simulink model "Degradation_Trial_1"  (R2022a)
settings: Solver=VariableStepAuto  StartTime=0.0  StopTime=500  RelTol=1e-3
libraries: nesl_utility x24, fl_lib x8
settings Model: Creator=YASH PATHAK  LastModifiedBy=YASH PATHAK

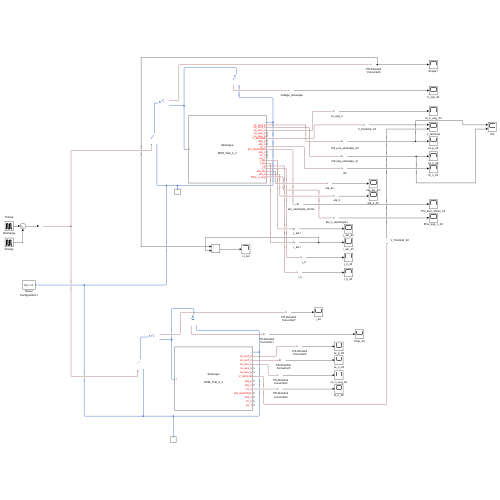
[thumbnail: Simulink's stored preview of the top-level diagram]
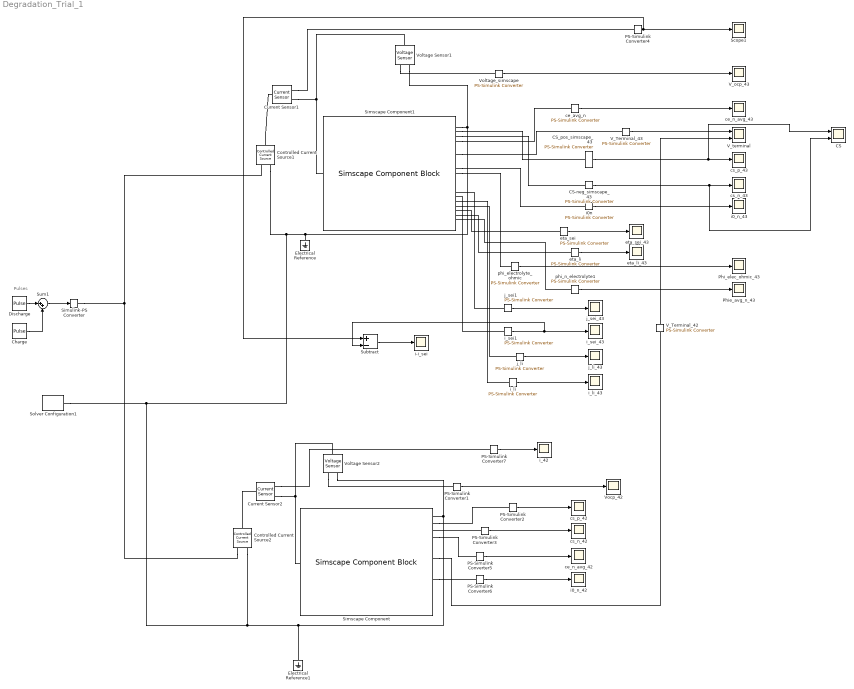
== system Degradation_Trial_1 ==
  note: Pulses
  CS : Scope  NumInputPorts=2
  CS-neg_simscape_43 : nesl_utility/PS-Simulink Converter  PhysicalDomain=network_engine_domain  SubClassName=ps_output  LeftPortType=input  RightPortType=output  PseudoPeriodic=off  Frequencies=[]  VectorFormat=inherit  Unit=inherit  AffineConversion=off
      settings: SourceProductBaseCode=SS,PW,VE
  CS_pos_simscape_43 : nesl_utility/PS-Simulink Converter  PhysicalDomain=network_engine_domain  SubClassName=ps_output  LeftPortType=input  RightPortType=output  PseudoPeriodic=off  Frequencies=[]  VectorFormat=inherit  Unit=inherit  AffineConversion=off
      settings: SourceProductBaseCode=SS,PW,VE
  Charge : DiscretePulseGenerator  PulseType=Time based  Amplitude=-25  Period=100  PulseWidth=25  PhaseDelay=75
  Controlled Current Source1 : fl_lib/Electrical/Electrical Sources/Controlled Current Source
      settings: SourceProductBaseCode=PW,SS,VE
  Controlled Current Source2 : fl_lib/Electrical/Electrical Sources/Controlled Current Source
      settings: SourceProductBaseCode=PW,SS,VE
  Current Sensor1 : fl_lib/Electrical/Electrical Sensors/Current Sensor
      settings: SourceProductBaseCode=PW,SS,VE
  Current Sensor2 : fl_lib/Electrical/Electrical Sensors/Current Sensor
      settings: SourceProductBaseCode=PW,SS,VE
  Discharge : DiscretePulseGenerator  PulseType=Time based  Amplitude=5  Period=100  PulseWidth=25  PhaseDelay=25
  Electrical Reference : fl_lib/Electrical/Electrical Elements/Electrical Reference
      settings: SourceProductBaseCode=PW,SS,VE
  Electrical Reference1 : fl_lib/Electrical/Electrical Elements/Electrical Reference
      settings: SourceProductBaseCode=PW,SS,VE
  PS-Simulink Converter{1..7} (7 alike) : nesl_utility/PS-Simulink Converter  PhysicalDomain=network_engine_domain  SubClassName=ps_output  LeftPortType=input  RightPortType=output  PseudoPeriodic=off  Frequencies=[]  VectorFormat=inherit  Unit=inherit  AffineConversion=off
      settings: SourceProductBaseCode=SS,PW,VE
  Phi_elec_ohmic_43 : Scope
  Phie_avg_n_43 : Scope
  Scope1 : Scope
  Simscape Component : SimscapeComponentBlock  SourceFile=SPM_Trial_4_2  ComponentPath=SPM_Trial_4_2  ComponentVariants="[\"SPM_Trial_4_2\"]"  ComponentVariantNames="[\"SPM_Trial_4_2\"]"  ClassName=SPM_Trial_4_2  SchemaVersion=1  nr=50  nn=50  ns=25  np=50  Rp=3.5e-06 m  Rn=2.5e-06 m  Ds_p=8e-15 m^2/s  Ds_n=5e-15 m^2/s  D_e=5.35e-10 m^2/s  D_e1=5.35e-10  SOC_0=0.1  brugg=1.5  t_plus=0.38  tf=0.62  ce_init=1000 mol/m^3  ce_init_unitless=1000  kappa=1.3 S/m  k0_n=1.061e-6 / 96485  k0_p=4.824e-6 / 96485  kt_n=1 * 0.0250 V*m^2/A  kt_p=0 * 300e-4 V*m^2/A  x100_percent_n=0.8292  x0_percent_n=3.5506e-04  y0_percent_p=0.8941  y100_percent_p=0.0335  del_p=6.7e-05 m  del_n=6.2e-05 m  del_s=1.2e-05 m  del_p1=6.7e-05  del_n1=6.2e-05  del_s1=1.2e-05  cs_max_p=35380 mol/m^3  cs_max_p_unitless=35380  cs_max_n=28746 mol/m^3  cs_max_n_unitless=28746  epsilon_e_p=0.3  epsilon_e_n=0.3  epsilon_e_s=0.4  Active_Area=0.205 m^2  Faradays=96485 C/mol  T=273.15 + 25  R=8.3145  Cap_n=6.0272 C  Cap_p=5.8050 C  i_specify=off  i_priority=None  i=0 A  i_nominal_specify=off  i_nominal_unit=A  i_nominal_value=1  v_specify=off  v_priority=None  v=0 V  v_nominal_specify=off  v_nominal_unit=V  v_nominal_value=1  UP_specify=off  UP_priority=None  UP=0  UP_nominal_specify=off  UP_nominal_unit=1  UP_nominal_value=1  UN_specify=off  UN_priority=None  UN=0  UN_nominal_specify=off  UN_nominal_unit=1  UN_nominal_value=1  V_ocp_specify=off  V_ocp_priority=None  V_ocp=0  V_ocp_nominal_specify=off  V_ocp_nominal_unit=1  V_ocp_nominal_value=1  j_n_specify=off  j_n_priority=None  j_n=0  j_n_nominal_specify=off  j_n_nominal_unit=1  j_n_nominal_value=1  j_p_specify=off  j_p_priority=None  j_p=0  j_p_nominal_specify=off  j_p_nominal_unit=1  j_p_nominal_value=1  i0_p_specify=off  i0_p_priority=None  i0_p=0  i0_p_nominal_specify=off  i0_p_nominal_unit=1  i0_p_nominal_value=1  Vr_p_specify=off  Vr_p_priority=None  Vr_p=0  Vr_p_nominal_specify=off  Vr_p_nominal_unit=1  Vr_p_nominal_value=1  x_specify=off  x_priority=None  x=0  x_nominal_specify=off  x_nominal_unit=1  x_nominal_value=1  y_specify=off  y_priority=None  y=0  y_nominal_specify=off  y_nominal_unit=1  y_nominal_value=1
      settings: CopyFcn=simscape.engine.sli.internal.componentblockcallback(gcbh,'COPY')  PreCopyFcn=simscape.engine.sli.internal.componentblockcallback(gcbh,'PRECOPY')  PreDeleteFcn=simscape.engine.sli.internal.componentblockcallback(gcbh,'PREDELETE')  InternalSimscapePortConfiguration="{\"Bottom\":[],\"Left\":[{\"id\":\"p\",\"label\":\"+\",\"type\":\"foundation.electrical.electrical\"}],\"Right\":[{\"id\":\"n\",\"label\":\"-\",\"type\":\"foundation.electrical.electrical\"},{\"id\":\"cs_surf_p\",\"label\":\"cs_surf_p\",\"type\":\"output\"},{\"id\":\"cs_surf_n\",\"label\":\"cs_surf_n\",\"type\":\"output\"},{\"id\":\"ce_ave_n\",\"label\":\"ce_ave_n\",\"type\":\"output\"},{\"id\":\"ce_ave_s\",\"label\":\"ce_ave_s\",\"type\":\"output\"},{\"id\":\"ce_ave_p\",\"label\":\"ce_ave_p\",\"type\":\"output\"},{\"id\":\"V_terminal\",\"label\":\"V_terminal\",\"type\":\"output\"},{\"id\":\"eta_p\",\"label\":\"eta_p\",\"type\":\"output\"},{\"id\":\"eta_n\",\"label\":\"eta_n\",\"type\":\"output\"},{\"id\":\"i0_n\",\"label\":\"i0_n\",\"type\":\"output\"},{\"id\":\"phi_electrolyte\",\"label\":\"phi_electrolyte\",\"type\":\"output\"},{\"id\":\"eta_c\",\"label\":\"eta_c\",\"type\":\"output\"},{\"id\":\"Vr_n\",\"label\":\"Vr_n\",\"type\":\"output\"},{\"id\":\"ce_1\",\"label\":\"ce_1\",\"type\":\"output\"}],\"Top\":[]}"
      mask Type: Two-port electrical component
  Simscape Component1 : SimscapeComponentBlock  SourceFile=SPM_Trial_4_3  ComponentPath=SPM_Trial_4_3  ComponentVariants="[\"SPM_Trial_4_3\"]"  ComponentVariantNames="[\"SPM_Trial_4_3\"]"  ClassName=SPM_Trial_4_3  SchemaVersion=1  nr=50  nn=50  ns=25  np=50  Rp=3.5e-06 m  Rn=2.5e-06 m  Ds_p=8e-15 m^2/s  Ds_n=5e-15 m^2/s  del_p=6.7e-05 m  del_n=6.2e-05 m  del_s=1.2e-05 m  del_p1=6.7e-05  del_n1=6.2e-05  del_s1=1.2e-05  cs_max_p=35380 mol/m^3  cs_max_p_unitless=35380  cs_max_n=28746 mol/m^3  cs_max_n_unitless=28746  epsilon_e_p=0.3  epsilon_e_n=0.3  epsilon_e_s=0.4  D_e=5.35e-10 m^2/s  D_e1=5.35e-10  brugg=1.5  t_plus=0.38  ce_init=1000 mol/m^3  ce_init_unitless=1000  kappa=1.3 S/m  k0_n=1.061e-6 / 96485  k0_p=4.824e-6 / 96485  kt_n=1 * 0.0250 V*m^2/A  kt_p=0 * 300e-4 V*m^2/A  x100_percent_n=0.8292  x0_percent_n=3.5506e-04  y0_percent_p=0.8941  y100_percent_p=0.0335  Faradays=96485 C/mol  T=273.15 + 25  R=8.3145  Cap_n=6.0272 C  Cap_p=5.8050 C  Active_Area=0.205 m^2  SOC_0=0.1  U_sei=0 V  i0pl=0.001 A/m^2  del_sei_init=5e-9 m  D_ec=2e-18 m^2/s  c_ec0=4541 mol/m^3  M_sei=0.162 kg/mol  rho_sei=1690 kg/m^3  k0_sei=1e-12 m/s  k_sei=5e-6 S/m  M_li=6.94e-3 kg/mol  rho_li=534 kg/m^3  i_specify=off  i_priority=None  i=0 A  i_nominal_specify=off  i_nominal_unit=A  i_nominal_value=1  v_specify=off  v_priority=None  v=0 V  v_nominal_specify=off  v_nominal_unit=V  v_nominal_value=1  UP_specify=off  UP_priority=None  UP=0  UP_nominal_specify=off  UP_nominal_unit=1  UP_nominal_value=1  UN_specify=off  UN_priority=None  UN=0  UN_nominal_specify=off  UN_nominal_unit=1  UN_nominal_value=1  V_ocp_specify=off  V_ocp_priority=None  V_ocp=0  V_ocp_nominal_specify=off  V_ocp_nominal_unit=1  V_ocp_nominal_value=1  Vr_p_specify=off  Vr_p_priority=None  Vr_p=0  Vr_p_nominal_specify=off  Vr_p_nominal_unit=1  Vr_p_nominal_value=1  j_n_specify=off  j_n_priority=None  j_n=0  j_n_nominal_specify=off  j_n_nominal_unit=1  j_n_nominal_value=1  j_p_specify=off  j_p_priority=None  j_p=0  j_p_nominal_specify=off  j_p_nominal_unit=1  j_p_nominal_value=1  i0_p_specify=off  i0_p_priority=None  i0_p=0  i0_p_nominal_specify=off  i0_p_nominal_unit=1  i0_p_nominal_value=1  x_specify=off  x_priority=None  x=0  x_nominal_specify=off  x_nominal_unit=1  x_nominal_value=1  y_specify=off  y_priority=None  y=0  y_nominal_specify=off  y_nominal_unit=1  y_nominal_value=1  Li_loss_specify=off  Li_loss_priority=None  Li_loss=0 mol  Li_loss_nominal_specify=off  Li_loss_nominal_unit=mol  Li_loss_nominal_value=1  Li_plated_specify=off  Li_plated_priority=None  Li_plated=0 mol  Li_plated_nominal_specify=off  Li_plated_nominal_unit=mol  Li_plated_nominal_value=1  Q_loss_specify=off  Q_loss_priority=None  Q_loss=0 A*hr  Q_loss_nominal_specify=off  Q_loss_nominal_unit=A*hr  Q_loss_nominal_value=1  soc_loss_specify=off  soc_loss_priority=None  soc_loss=0  soc_loss_nominal_specify=off  soc_loss_nominal_unit=1  soc_loss_nominal_value=1
      settings: CopyFcn=simscape.engine.sli.internal.componentblockcallback(gcbh,'COPY')  PreCopyFcn=simscape.engine.sli.internal.componentblockcallback(gcbh,'PRECOPY')  PreDeleteFcn=simscape.engine.sli.internal.componentblockcallback(gcbh,'PREDELETE')  InternalSimscapePortConfiguration="{\"Bottom\":[],\"Left\":[{\"id\":\"p\",\"label\":\"+\",\"type\":\"foundation.electrical.electrical\"}],\"Right\":[{\"id\":\"n\",\"label\":\"-\",\"type\":\"foundation.electrical.electrical\"},{\"id\":\"cs_surf_p\",\"label\":\"cs_surf_p\",\"type\":\"output\"},{\"id\":\"cs_surf_n\",\"label\":\"cs_surf_n\",\"type\":\"output\"},{\"id\":\"ce_ave_n\",\"label\":\"ce_ave_n\",\"type\":\"output\"},{\"id\":\"ce_ave_s\",\"label\":\"ce_ave_s\",\"type\":\"output\"},{\"id\":\"ce_ave_p\",\"label\":\"ce_ave_p\",\"type\":\"output\"},{\"id\":\"V_terminal\",\"label\":\"V_terminal\",\"type\":\"output\"},{\"id\":\"eta_p\",\"label\":\"eta_p\",\"type\":\"output\"},{\"id\":\"eta_n\",\"label\":\"eta_n\",\"type\":\"output\"},{\"id\":\"i0_n\",\"label\":\"i0_n\",\"type\":\"output\"},{\"id\":\"phi_electrolyte\",\"label\":\"phi_electrolyte\",\"type\":\"output\"},{\"id\":\"eta_c\",\"label\":\"eta_c\",\"type\":\"output\"},{\"id\":\"Vr_n\",\"label\":\"Vr_n\",\"type\":\"output\"},{\"id\":\"ce_1\",\"label\":\"ce_1\",\"type\":\"output\"},{\"id\":\"j_sei\",\"label\":\"j_sei\",\"type\":\"output\"},{\"id\":\"i_sei\",\"label\":\"i_sei\",\"type\":\"output\"},{\"id\":\"i_li\",\"label\":\"i_li\",\"type\":\"output\"},{\"id\":\"j_li\",\"label\":\"j_li\",\"type\":\"output\"},{\"id\":\"eta_sei\",\"label\":\"eta_sei\",\"type\":\"output\"},{\"id\":\"eta_li\",\"label\":\"eta_li\",\"type\":\"output\"},{\"id\":\"Phie_n_avg\",\"label\":\"Phie_n_avg\",\"type\":\"output\"}],\"Top\":[]}"
      mask Type: Two-port electrical component
  Simulink-PS Converter : nesl_utility/Simulink-PS Converter  PhysicalDomain=network_engine_domain  SubClassName=ps_input  LeftPortType=input  RightPortType=output  PseudoPeriodic=off  Frequencies=[]  NoiseDistribution=none  NoiseParameters=[]  Unit=1  AffineConversion=off  FilteringAndDerivatives=provide  SimscapeFilterOrder=1  InputFilterTimeConstant=0.001  UdotUserProvided=0
      settings: SourceProductBaseCode=SS,PW,VE
  Solver Configuration1 : nesl_utility/Solver Configuration  PhysicalDomain=network_engine_domain  SubClassName=solver  LeftPortType=input  RightPortType=generic  Tones=[]  Harmonics=[]  SimulateNoise=off  Profile=off  UseLocalSampling=off  EnableSwitchedLinearOptims=on  FrequencyDomain=off  UseCCode=off  RelTol=0.001  AbsTol=1e-06  MinStep=1e-09  ToWorkspace=off  RevertToSquareIcSolve=off  NumHomotopyIterations=100  PhasorMode=off  PhasorModeNumHarmonics=1  IndexReductionMethod=DerivativeReplacement  DoDC=off  ResidualTolerance=1e-09  UseLocalSolver=off  LocalSolverChoice=NE_BACKWARD_EULER_ADVANCER  LocalSolverSampleTime=0.001  DoFixedCost=off  MaxNonlinIter=3  MaxModeIter=2  ComputeImpulses=off  ImpulseIterations=2  LinearAlgebra=auto  LinearAlgebraNumThread=0  EquationFormulation=NE_TIME_EF  DelaysMemoryBudget=1024  AutomaticFiltering=on  FilteringTimeConstant=0.001  PartitionStorageMethod=AS_NEEDED  PartitionMemoryBudget=1024  PartitionMethod=ROBUST
      settings: SourceProductBaseCode=SS,PW,VE
  Subtract : Sum  Inputs=+-
  Sum1 : Sum  Inputs=|++
  V_Terminal_42 : nesl_utility/PS-Simulink Converter  PhysicalDomain=network_engine_domain  SubClassName=ps_output  LeftPortType=input  RightPortType=output  PseudoPeriodic=off  Frequencies=[]  VectorFormat=inherit  Unit=inherit  AffineConversion=off
      settings: SourceProductBaseCode=SS,PW,VE
  V_Terminal_43 : nesl_utility/PS-Simulink Converter  PhysicalDomain=network_engine_domain  SubClassName=ps_output  LeftPortType=input  RightPortType=output  PseudoPeriodic=off  Frequencies=[]  VectorFormat=inherit  Unit=inherit  AffineConversion=off
      settings: SourceProductBaseCode=SS,PW,VE
  V_ocp_43 : Scope
  V_terminal : Scope  NumInputPorts=2
  Vocp_42 : Scope
  Voltage Sensor1 : fl_lib/Electrical/Electrical Sensors/Voltage Sensor
      settings: SourceProductBaseCode=PW,SS,VE
  Voltage Sensor2 : fl_lib/Electrical/Electrical Sensors/Voltage Sensor
      settings: SourceProductBaseCode=PW,SS,VE
  Voltage_simscape : nesl_utility/PS-Simulink Converter  PhysicalDomain=network_engine_domain  SubClassName=ps_output  LeftPortType=input  RightPortType=output  PseudoPeriodic=off  Frequencies=[]  VectorFormat=inherit  Unit=inherit  AffineConversion=off
      settings: SourceProductBaseCode=SS,PW,VE
  ce_avg_n : nesl_utility/PS-Simulink Converter  PhysicalDomain=network_engine_domain  SubClassName=ps_output  LeftPortType=input  RightPortType=output  PseudoPeriodic=off  Frequencies=[]  VectorFormat=inherit  Unit=inherit  AffineConversion=off
      settings: SourceProductBaseCode=SS,PW,VE
  ce_n_avg_42 : Scope
  ce_n_avg_43 : Scope
  cs_n_42 : Scope
  cs_n_43 : Scope
  cs_p_42 : Scope
  cs_p_43 : Scope
  eta_li : nesl_utility/PS-Simulink Converter  PhysicalDomain=network_engine_domain  SubClassName=ps_output  LeftPortType=input  RightPortType=output  PseudoPeriodic=off  Frequencies=[]  VectorFormat=inherit  Unit=inherit  AffineConversion=off
      settings: SourceProductBaseCode=SS,PW,VE
  eta_li_43 : Scope
  eta_sei : nesl_utility/PS-Simulink Converter  PhysicalDomain=network_engine_domain  SubClassName=ps_output  LeftPortType=input  RightPortType=output  PseudoPeriodic=off  Frequencies=[]  VectorFormat=inherit  Unit=inherit  AffineConversion=off
      settings: SourceProductBaseCode=SS,PW,VE
  eta_sei_43 : Scope
  i-i_sei : Scope
  i0_n_42 : Scope
  i0_n_43 : Scope
  i0n : nesl_utility/PS-Simulink Converter  PhysicalDomain=network_engine_domain  SubClassName=ps_output  LeftPortType=input  RightPortType=output  PseudoPeriodic=off  Frequencies=[]  VectorFormat=inherit  Unit=inherit  AffineConversion=off
      settings: SourceProductBaseCode=SS,PW,VE
  i_42 : Scope
  i_li : nesl_utility/PS-Simulink Converter  PhysicalDomain=network_engine_domain  SubClassName=ps_output  LeftPortType=input  RightPortType=output  PseudoPeriodic=off  Frequencies=[]  VectorFormat=inherit  Unit=inherit  AffineConversion=off
      settings: SourceProductBaseCode=SS,PW,VE
  i_li_43 : Scope
  i_sei1 : nesl_utility/PS-Simulink Converter  PhysicalDomain=network_engine_domain  SubClassName=ps_output  LeftPortType=input  RightPortType=output  PseudoPeriodic=off  Frequencies=[]  VectorFormat=inherit  Unit=inherit  AffineConversion=off
      settings: SourceProductBaseCode=SS,PW,VE
  i_sei_43 : Scope
  j_li : nesl_utility/PS-Simulink Converter  PhysicalDomain=network_engine_domain  SubClassName=ps_output  LeftPortType=input  RightPortType=output  PseudoPeriodic=off  Frequencies=[]  VectorFormat=inherit  Unit=inherit  AffineConversion=off
      settings: SourceProductBaseCode=SS,PW,VE
  j_li_43 : Scope
  j_sei1 : nesl_utility/PS-Simulink Converter  PhysicalDomain=network_engine_domain  SubClassName=ps_output  LeftPortType=input  RightPortType=output  PseudoPeriodic=off  Frequencies=[]  VectorFormat=inherit  Unit=inherit  AffineConversion=off
      settings: SourceProductBaseCode=SS,PW,VE
  j_sei_43 : Scope
  phi_electrolyte_ohmic : nesl_utility/PS-Simulink Converter  PhysicalDomain=network_engine_domain  SubClassName=ps_output  LeftPortType=input  RightPortType=output  PseudoPeriodic=off  Frequencies=[]  VectorFormat=inherit  Unit=inherit  AffineConversion=off
      settings: SourceProductBaseCode=SS,PW,VE
  phi_n_electrolyte1 : nesl_utility/PS-Simulink Converter  PhysicalDomain=network_engine_domain  SubClassName=ps_output  LeftPortType=input  RightPortType=output  PseudoPeriodic=off  Frequencies=[]  VectorFormat=inherit  Unit=inherit  AffineConversion=off
      settings: SourceProductBaseCode=SS,PW,VE
  wires:
  PS-Simulink Converter4/1 -> Scope1/1, Subtract/1
  Voltage_simscape/1 -> V_ocp_43/1
  CS-neg_simscape_43/1 -> CS/2, cs_n_43/1
  CS_pos_simscape_43/1 -> CS/1, cs_p_43/1
  i0n/1 -> i0_n_43/1
  ce_avg_n/1 -> ce_n_avg_43/1
  phi_electrolyte_ohmic/1 -> Phi_elec_ohmic_43/1
  j_li/1 -> j_li_43/1
  j_sei1/1 -> j_sei_43/1
  i_sei1/1 -> Subtract/2, i_sei_43/1
  i_li/1 -> i_li_43/1
  eta_sei/1 -> eta_sei_43/1
  eta_li/1 -> eta_li_43/1
  phi_n_electrolyte1/1 -> Phie_avg_n_43/1
  V_Terminal_43/1 -> V_terminal/1
  PS-Simulink Converter1/1 -> Vocp_42/1
  PS-Simulink Converter2/1 -> cs_p_42/1
  PS-Simulink Converter3/1 -> cs_n_42/1
  PS-Simulink Converter5/1 -> ce_n_avg_42/1
  PS-Simulink Converter6/1 -> i0_n_42/1
  V_Terminal_42/1 -> V_terminal/2
  Subtract/1 -> i-i_sei/1
  PS-Simulink Converter7/1 -> i_42/1
  Discharge/1 -> Sum1/1
  Sum1/1 -> Simulink-PS Converter/1
  Charge/1 -> Sum1/2
  connections:
  Current Sensor1/RConn2 -- Simscape Component1/LConn1 -- Voltage Sensor1/LConn1
  Simscape Component1/RConn3 -- CS-neg_simscape_43/LConn1
  Simscape Component1/RConn2 -- CS_pos_simscape_43/LConn1
  Voltage Sensor1/RConn1 -- Voltage_simscape/LConn1
  Current Sensor1/RConn1 -- PS-Simulink Converter4/LConn1
  Simscape Component1/RConn10 -- i0n/LConn1
  Simscape Component1/RConn4 -- ce_avg_n/LConn1
  Simscape Component1/RConn11 -- phi_electrolyte_ohmic/LConn1
  j_sei1/LConn1 -- Simscape Component1/RConn15
  j_li/LConn1 -- Simscape Component1/RConn18
  i_sei1/LConn1 -- Simscape Component1/RConn16
  eta_sei/LConn1 -- Simscape Component1/RConn19
  eta_li/LConn1 -- Simscape Component1/RConn20
  phi_n_electrolyte1/LConn1 -- Simscape Component1/RConn21
  Simscape Component1/RConn7 -- V_Terminal_43/LConn1
  Voltage Sensor2/LConn1 -- Current Sensor2/RConn2 -- Simscape Component/LConn1
  Voltage Sensor1/RConn2 -- Simscape Component1/RConn1 -- Controlled Current Source1/RConn2 -- Controlled Current Source2/RConn2 -- Electrical Reference1/LConn1 -- Voltage Sensor2/RConn2 -- Simscape Component/RConn1 -- Solver Configuration1/RConn1 -- Electrical Reference/LConn1
  Voltage Sensor2/RConn1 -- PS-Simulink Converter1/LConn1
  Simscape Component/RConn2 -- PS-Simulink Converter2/LConn1
  PS-Simulink Converter3/LConn1 -- Simscape Component/RConn3
  Simscape Component/RConn4 -- PS-Simulink Converter5/LConn1
  Simscape Component/RConn10 -- PS-Simulink Converter6/LConn1
  Simscape Component/RConn7 -- V_Terminal_42/LConn1
  Current Sensor2/RConn1 -- PS-Simulink Converter7/LConn1
  Simscape Component1/RConn17 -- i_li/LConn1
  Simulink-PS Converter/RConn1 -- Controlled Current Source1/RConn1 -- Controlled Current Source2/RConn1
  Controlled Current Source1/LConn1 -- Current Sensor1/LConn1
  Controlled Current Source2/LConn1 -- Current Sensor2/LConn1
